simulink model "rtwdemo_paraminline"  (Simulink 6.0)
settings: Solver=FixedStepDiscrete  StartTime=0.0  StopTime=10.0  RelTol=1e-3
PreLoadFcn:
  | rtwdemo_paraminline_data
values from neighbouring files (symbols this model uses):
  MAX_LIFT = Simulink.Parameter    [rtwdemo_paraminline_data.m]
  SLIDER_POS = Simulink.Parameter    [rtwdemo_paraminline_data.m]
  T1Break = Simulink.Parameter    [rtwdemo_exprfolding_data.m]    (also in rtwdemo_paraminline_data.m; rtwdemo_ssreuse_data.m)
  T1Data = Simulink.Parameter    [rtwdemo_exprfolding_data.m]    (also in rtwdemo_paraminline_data.m; rtwdemo_ssreuse_data.m)
  T2Data = Simulink.Parameter    [rtwdemo_exprfolding_data.m]    (also in rtwdemo_paraminline_data.m; rtwdemo_ssreuse_data.m = copy(T1Data))
libraries: rtwdemowidgets x3
settings Model: CovMetricSettings=d  Creator=The MathWorks Inc.  LastModifiedBy=batserve  ExtModeAutoUpdateStatusClock=off
settings DataIOCC: SaveOutput=off  SaveTime=off  SignalLoggingName=sigsOut
settings OptimizationCC: InlineParams=on  EnforceIntegerDowncast=off  StateBitsets=on  DataBitsets=on  UseTempVars=on
settings DebuggingCC: CheckExecutionContextPreStartOutputMsg=on  CheckExecutionContextRuntimeOutputMsg=on  SignalResolutionControl=UseLocalSettings  SolverPrmCheckMsg=none
settings RTWCC: TLCOptions=-p0 -aWarnNonSaturatedBlocks=0  GenCodeOnly=on  GenerateReport=on  RTWVerbose=off  ProcessScript=grt_make_rtw_hook  LaunchReport=on
settings CodeAppCC: ForceParamTrailComments=on  PrefixModelToSubsysFcnNames=off
settings GRTTargetCC: MatFileLogging=off

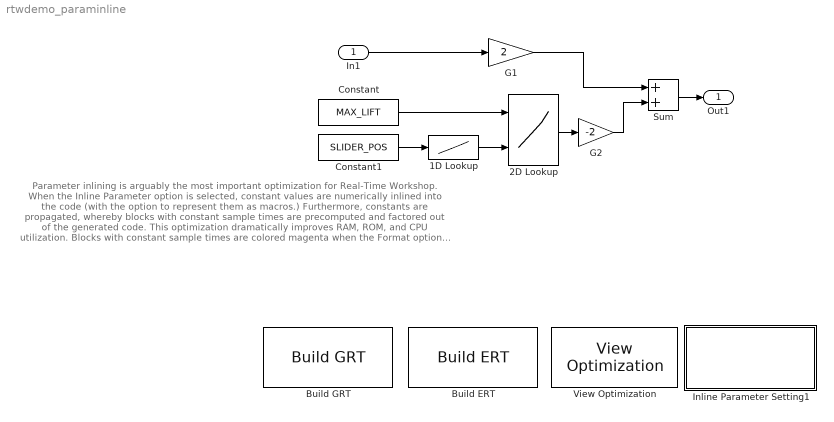
== system rtwdemo_paraminline ==
  note: Parameter inlining is arguably the most important optimization for Real-Time Workshop.  When the
      | Inline Parameter option is selected, constant values are numerically inlined into the code (with
      | the option to represent them as macros.)  Furthermore, constants are propagated, whereby blocks
      | with constant sample times are precomputed and factored out of the generated code.  This
      | optimization dramatically improves RAM, ROM, and CPU utilization.  Blocks with constant sample
      | times are colored magenta when the Format option 'Sample Time Colors' is selected.
  In1 : Inport  Port=1  PortDimensions=1  LatchInput=off
  1D Lookup : Lookup  DialogController=Simulink.DDGSource  InputValues=T1Break  OutputValues=T1Data  SaturateOnIntegerOverflow=on
  2D Lookup : Lookup2D  DialogController=Simulink.DDGSource  RowIndex=T2Break  ColumnIndex=T2Break  OutputValues=T2Data  OutScaling=2^-10  InputSameDT=on
  Build ERT : rtwdemowidgets/Build ERT  attrib_overrides={}
  Build GRT : rtwdemowidgets/Build GRT  attrib_overrides={}
  Constant : Constant  Value=MAX_LIFT
  Constant1 : Constant  Value=SLIDER_POS
  G1 : Gain  Gain=2  SaturateOnIntegerOverflow=on
  G2 : Gain  Gain=-2  SaturateOnIntegerOverflow=on
  Inline Parameter Setting1 : Subsystem  Orientation=up  PropExecContextAcrossSSBoundary=on
      settings: OpenFcn=m=get_param(bdroot,'name'); eval([m,'([],[],[],''compile'');']); eval([m,'([],[],[],''term'');']);
      mask Display: disp(sprintf('Display Sample\nTime Colors\n(double-click)'))
  Sum : Sum  OutScaling=2^-10
  View Optimization : rtwdemowidgets/View Optimization
  Out1 : Outport
  wires:
  In1/1 -> G1/1
  Sum/1 -> Out1/1
  Constant/1 -> 2D Lookup/1
  Constant1/1 -> 1D Lookup/1
  1D Lookup/1 -> 2D Lookup/2
  2D Lookup/1 -> G2/1
  G1/1 -> Sum/1
  G2/1 -> Sum/2

== system rtwdemo_paraminline/Inline Parameter Setting1 ==
